simulink model "LF_AC29bus_HVDCdemo_V2_1"  (R2019b)
settings: Solver=FixedStepDiscrete  StartTime=0.0  StopTime=fix(6/Ts)*Ts  FixedStep=Ts  RelTol=1e-3
InitFcn:
  | Ts_avg=150e-6;
  | Ts=50e-6;
  | 
  | %Tc_stab = 1/60/5;
  | %Tc_stab = 2/60;
  | Tc_stab = Ts;
  | 
  | 
  | Ts_avg=150e-6;
  | 
  | Ts=50e-6;
  | 
  | % Rectifier AC side :
  | VLL_nom_R = 735e3; % V
  | Fnom_R = 60;           % Hz
  | 
  | % Inverter AC side :
  | VLL_nom_I = 735e3; % V
  | Fnom_I = 60;           % Hz
  | 
  | % DC :
  | Vdc_nom = 500e3;   % V
  | Idc_nom  = 2000;     % A
undefined symbols (not defined in the file): D1, D11, Delta, test_alpha
libraries: powerlib x223, powerlib_meascontrol x57, simulink x22, sps_avr x7
(part 2 of 10)

== system LF_AC29bus_HVDCdemo_V2_1/HVDC_network_avg ==
  note: HVDC 12-pulse Transmission System 1000 MW (500kV-2kA) 60 Hz (Average Model)
  Binv : powerlib/Measurements/Three-Phase V-I Measurement  VoltageMeasurement=phase-to-ground  SetLabelV=on  LabelV=Vabc_I  Vpu=on  VpuLL=off  CurrentMeasurement=yes  SetLabelI=on  LabelI=Iabc_I  Ipu=on  Pbase=100e6  Vbase=735e3  OutputType=Magnitude  PhasorSimulation=off  PSBequivalent=0
      settings: SourceProductName=Simscape Electrical
  Brect : powerlib/Measurements/Three-Phase V-I Measurement  VoltageMeasurement=phase-to-ground  SetLabelV=on  LabelV=Vabc_R  Vpu=on  VpuLL=off  CurrentMeasurement=yes  SetLabelI=on  LabelI=Iabc_R  Ipu=on  Pbase=100e6  Vbase=735e3  OutputType=Magnitude  PhasorSimulation=off  PSBequivalent=0
      settings: SourceProductName=Simscape Electrical
  DC line 800 km : powerlib/Elements/Distributed Parameters Line  Phases=1  Frequency=60  Resistance=0.015  Inductance=0.792e-3  Capacitance=14.4e-9  Length=800  x1=[-0.00275 0;-0.0027 0;-0.00265 0;-0.0026 0;-0.00255 0;-0.0025 0;-0.00245 0;-0.0024 0;-0.00235 0;-0.0023 0;-0.00225 0;-0.0022 0;-0.00215 0;-0.0021 0;-0.00205 0;-0.002 0;-0.00195 0;-0.0019 0;-0.00185 0;-0.0018 0;-0.00175 0;-0.0017 0;-0.00165 0;-0.0016 0;-0.00155 0;-0.0015 0;-0.00145 0;-0.0014 0;-0.00135 0;-0.0013 0;-0.00125 0;-0.0012 0;-0.00115 0;-0.0011 0;-0.00105 0;-0.001 0;-0.00095 0;-0.0009 0;-0.00085 0;-0.0008 0;-0.00075 0;-0.0007 0;-0.00065 0;-0.0006 0;-0.00055 0;-0.0005 0;-0.00045 0;-0.0004 0;-0.00035 0;-0.0003 0;-0.00025 0;-0.0002 0;-0.00015 0;-0.0001 0;-5e-05 0]  x2=[-0.00275 0;-0.0027 0;-0.00265 0;-0.0026 0;-0.00255 0;-0.0025 0;-0.00245 0;-0.0024 0;-0.00235 0;-0.0023 0;-0.00225 0;-0.0022 0;-0.00215 0;-0.0021 0;-0.00205 0;-0.002 0;-0.00195 0;-0.0019 0;-0.00185 0;-0.0018 0;-0.00175 0;-0.0017 0;-0.00165 0;-0.0016 0;-0.00155 0;-0.0015 0;-0.00145 0;-0.0014 0;-0.00135 0;-0.0013 0;-0.00125 0;-0.0012 0;-0.00115 0;-0.0011 0;-0.00105 0;-0.001 0;-0.00095 0;-0.0009 0;-0.00085 0;-0.0008 0;-0.00075 0;-0.0007 0;-0.00065 0;-0.0006 0;-0.00055 0;-0.0005 0;-0.00045 0;-0.0004 0;-0.00035 0;-0.0003 0;-0.00025 0;-0.0002 0;-0.00015 0;-0.0001 0;-5e-05 0]  x3=[-0.00275 0;-0.0027 0;-0.00265 0;-0.0026 0;-0.00255 0;-0.0025 0;-0.00245 0;-0.0024 0;-0.00235 0;-0.0023 0;-0.00225 0;-0.0022 0;-0.00215 0;-0.0021 0;-0.00205 0;-0.002 0;-0.00195 0;-0.0019 0;-0.00185 0;-0.0018 0;-0.00175 0;-0.0017 0;-0.00165 0;-0.0016 0;-0.00155 0;-0.0015 0;-0.00145 0;-0.0014 0;-0.00135 0;-0.0013 0;-0.00125 0;-0.0012 0;-0.00115 0;-0.0011 0;-0.00105 0;-0.001 0;-0.00095 0;-0.0009 0;-0.00085 0;-0.0008 0;-0.00075 0;-0.0007 0;-0.00065 0;-0.0006 0;-0.00055 0;-0.0005 0;-0.00045 0;-0.0004 0;-0.00035 0;-0.0003 0;-0.00025 0;-0.0002 0;-0.00015 0;-0.0001 0;-5e-05 0]  x4=[-0.00275 0;-0.0027 0;-0.00265 0;-0.0026 0;-0.00255 0;-0.0025 0;-0.00245 0;-0.0024 0;-0.00235 0;-0.0023 0;-0.00225 0;-0.0022 0;-0.00215 0;-0.0021 0;-0.00205 0;-0.002 0;-0.00195 0;-0.0019 0;-0.00185 0;-0.0018 0;-0.00175 0;-0.0017 0;-0.00165 0;-0.0016 0;-0.00155 0;-0.0015 0;-0.00145 0;-0.0014 0;-0.00135 0;-0.0013 0;-0.00125 0;-0.0012 0;-0.00115 0;-0.0011 0;-0.00105 0;-0.001 0;-0.00095 0;-0.0009 0;-0.00085 0;-0.0008 0;-0.00075 0;-0.0007 0;-0.00065 0;-0.0006 0;-0.00055 0;-0.0005 0;-0.00045 0;-0.0004 0;-0.00035 0;-0.0003 0;-0.00025 0;-0.0002 0;-0.00015 0;-0.0001 0;-5e-05 0]  x5=0.0027016794776583  V1=ones(3,3)  V2=ones(3,3)  I1=ones(3,3)  I2=ones(3,3)  nHarmo=1  Measurements=Phase-to-ground voltages
      settings: AttributesFormatString=\n  SourceProductName=Simscape Electrical
  Filters 60Hz1 : Subsystem
      mask Display: disp('AC filters \n60 Hz\n600 Mvar')
  Filters 60Hz2 : Subsystem
      mask Display: disp('AC filters \n60 Hz\n600 Mvar')
  Ground1 : powerlib/Elements/Ground  LConnTagsString=a
      settings: SourceProductName=Simscape Electrical
  Ground4 : powerlib/Elements/Ground  LConnTagsString=a
      settings: SourceProductName=Simscape Electrical
  Inverter Average model : Subsystem
  Inverter Control and Protection (Average model) : Subsystem
      mask Display: disp('Pole Control\n and Protection')
  Ld1 : powerlib/Elements/Series RLC Branch  LConnTagsString=__new0  RConnTagsString=__new0  BranchType=RL  Resistance=0.3  Inductance=0.5  SetiL0=off  InitialCurrent=0  Capacitance=1.0  Setx0=off  InitialVoltage=0  Measurements=None
      settings: AttributesFormatString=%<Resistance> (ohm), %<Inductance> (H)  SourceProductName=Simscape Electrical
  Ld2 : powerlib/Elements/Series RLC Branch  LConnTagsString=__new0  RConnTagsString=__new0  BranchType=RL  Resistance=0.3  Inductance=0.5  SetiL0=off  InitialCurrent=0  Capacitance=1.0  Setx0=off  InitialVoltage=0  Measurements=None
      settings: AttributesFormatString=%<Resistance> (ohm), %<Inductance> (H)  SourceProductName=Simscape Electrical
  Master Control : Subsystem
      mask Display: disp('Master Control')
  Rectifier Average model : Subsystem
  Rectifier Control and Protection (Average model) : Subsystem
      mask Display: disp('Pole Control\n and Protection')
  A : PMIOPort  Tag=PMCPort  Side=Left
  B : PMIOPort  Tag=PMCPort  Port=2  Side=Left
  C : PMIOPort  Tag=PMCPort  Port=3  Side=Left
  "A " : PMIOPort  Tag=PMCPort  Port=4  Side=Right
  "B " : PMIOPort  Tag=PMCPort  Port=5  Side=Right
  "C " : PMIOPort  Tag=PMCPort  Port=6  Side=Right
  connections:
  Ld2/RConn1 -- Inverter Average model/RConn1
  Ld1/RConn1 -- DC line 800 km/LConn1
  Ld1/LConn1 -- Rectifier Average model/RConn1
  Ld2/LConn1 -- DC line 800 km/RConn1
  Ground1/LConn1 -- Inverter Average model/RConn2
  Inverter Average model/LConn1 -- Binv/RConn1
  Inverter Average model/LConn2 -- Binv/RConn2
  Inverter Average model/LConn3 -- Binv/RConn3
  Brect/RConn1 -- Rectifier Average model/LConn1
  Brect/RConn2 -- Rectifier Average model/LConn2
  Brect/RConn3 -- Rectifier Average model/LConn3
  Rectifier Average model/RConn2 -- Ground4/LConn1
  Brect/LConn2 -- B/RConn1 -- Filters 60Hz1/LConn2
  Brect/LConn1 -- A/RConn1 -- Filters 60Hz1/LConn1
  Brect/LConn3 -- C/RConn1 -- Filters 60Hz1/LConn3
  "A "/RConn1 -- Binv/LConn1 -- Filters 60Hz2/LConn1
  "B "/RConn1 -- Binv/LConn2 -- Filters 60Hz2/LConn2
  "C "/RConn1 -- Binv/LConn3 -- Filters 60Hz2/LConn3

== system LF_AC29bus_HVDCdemo_V2_1/LG27_nodes ==
  Neutral : powerlib/Elements/Neutral  LConnTagsString=a  NodeNumber=4
      settings: SourceProductName=Simscape Electrical  SourceProductBaseCode=PS
  Neutral1 : powerlib/Elements/Neutral  LConnTagsString=a  NodeNumber=5
      settings: SourceProductName=Simscape Electrical  SourceProductBaseCode=PS
  Neutral2 : powerlib/Elements/Neutral  LConnTagsString=a  NodeNumber=6
      settings: SourceProductName=Simscape Electrical  SourceProductBaseCode=PS
  a : PMIOPort  Tag=PMCPort  Side=Left
  b : PMIOPort  Tag=PMCPort  Port=2  Side=Left
  c : PMIOPort  Tag=PMCPort  Port=3  Side=Left
  connections:
  c/RConn1 -- Neutral2/LConn1
  b/RConn1 -- Neutral1/LConn1
  a/RConn1 -- Neutral/LConn1

== system LF_AC29bus_HVDCdemo_V2_1/MTL Load ==
  note: Constant PQ
  note: Constant Z
  note: TOTAL LOAD = 15 500 MW
  22 000 MVA 735 kV/230 kV : powerlib/Elements/Three-Phase Transformer (Two Windings)  Winding1Connection=Yg  Winding2Connection=Delta (D1)  CoreType=Three single-phase transformers  SetSaturation=off  Hysteresis=off  DataFile='basic_model'  SetInitialFlux=off  Measurements=None  UNITS=pu  NominalPower=[ 22000e6 60 ]  Winding1="[ 735e3 0.002  0.12]"  Winding2=[230e3 0.002 0]  Rm=500  Lm=500  L0=0.5  Saturation="[ 0,0  ;  0.005,1.2  ;  1.0,1.4 ]"  InitialFluxes=[ 0.8 , -0.8 , 0.7 ]  BreakLoop=off  DiscreteSolver=Trapezoidal iterative  DataType=off  TransfoNumber=0
      settings: SourceProductName=Simscape Electrical
  230 kV/25 kV 18 000 MVA : powerlib/Elements/Three-Phase Transformer (Two Windings)  Winding1Connection=Yg  Winding2Connection=Delta (D1)  CoreType=Three single-phase transformers  SetSaturation=off  Hysteresis=off  DataFile='basic_model'  SetInitialFlux=off  Measurements=None  UNITS=pu  NominalPower=[18000e6 60 ]  Winding1="[ 230e3  0.08/30   0.08 ]"  Winding2="[ 25e3  0.08/30  0.08]"  Rm=500  Lm=500  L0=0.5  Saturation="[ 0,0  ;  0.005,1.2  ;  1.0,1.4 ]"  InitialFluxes=[ 0.8 , -0.8 , 0.7 ]  BreakLoop=off  DiscreteSolver=Trapezoidal iterative  DataType=off  TransfoNumber=0
      settings: SourceProductName=Simscape Electrical
  3500 MW : powerlib/Elements/Three-Phase Dynamic Load  NominalVoltage=[ 25e3 60 ]  ActiveReactivePowers=[3.5e+09 -2.66454e-07]  PositiveSequence=[1.013 -91.543]  ExternalControl=off  NpNq="[1.5  2.5]"  TimeConstants="[0  0  0  0]"  MinimumVoltage=0.7  Tfilter=1e-4  LoadFlowParameters=[4,0,0,0,0]
      settings: SourceProductName=Simscape Electrical  SourceProductBaseCode=PS
  ASM 25kV 5000MVA Pm=4000 MW : powerlib/Machines/Asynchronous Machine pu Units  RotorType=Squirrel-cage  PresetModel=No  MechanicalLoad=Torque Tm  ShowDetailedParameters=on  ReferenceFrame=Rotor  Units=pu  MeasurementBus=off  NominalParameters="[5000e6 25e3  60]"  Stator=[0.01117 0.04832]  Rotor=[0.006 0.04832]  Cage1=[0.01909 0.0397]  Cage2=[0.01909 0.0397]  Lm=2.424  Mechanical="[1  0   2]"  PolePairs=2  InitialConditions=[0.00500983 0 0.928577 0.928577 0.928577 -121.661 -241.661 -1.66098]  SimulateSaturation=off  Saturation="[0.212,0.4201,0.8125,1.0979,1.4799,2.2457,3.2586,4.5763,6.4763 ;   0.5,0.7,0.9,1,1.1,1.2 ,1.3,1.4,1.5]"  LoadFlowParameters=0  TsPowergui=0  TsBlock=-1  IterativeModel=Trapezoidal non iterative  IterativeDiscreteModel=Trapezoidal non iterative  Pmec=4000e6
      settings: SourceProductName=Simscape Electrical  SourceProductBaseCode=PS
  Load Flow Bus : powerlib/Measurements/Load Flow Bus  LConnTagsString=a  Phases=single  Connectors=on one side  ID=MTL2  Vbase=230e3  Vref=1  Vangle=0  VLF=1.03  VLFb=1  VLFc=1  angleLF=-53.86  angleLFb=0  angleLFc=0
      settings: AttributesFormatString=%<ID>\n%<Vbase>V\n%<VLF>pu\n%<angleLF>deg.  SourceProductName=Simscape Electrical
  Load Flow Bus1 : powerlib/Measurements/Load Flow Bus  LConnTagsString=a  Phases=single  Connectors=on one side  ID=MTL_25  Vbase=25e3  Vref=1  Vangle=0  VLF=1.013  VLFb=1  VLFc=1  angleLF=-91.54  angleLFb=0  angleLFc=0
      settings: AttributesFormatString=%<ID>\n%<Vbase>V\n%<VLF>pu\n%<angleLF>deg.  SourceProductName=Simscape Electrical
  MTL 2000 Mvar : powerlib/Elements/Three-Phase Parallel RLC Load  LConnTagsString=A|B|C  Configuration=Y (grounded)  NominalVoltage=25e3  Vabc=[1e3 1e3 1e3]  Vabcp=[1e3 1e3 1e3]  NominalFrequency=60  UnbalancedPower=off  ActivePower=0  InductivePower=0  CapacitivePower=2000e6  Pabc=[10e3 9e3 11e3]  QLabc=[100 90 110]  QCabc=[100 90 110]  Pabcp=[10e3 9e3 11e3]  QLabcp=[100 90 110]  QCabcp=[100 90 110]  Measurements=None  LoadType=constant Z
      settings: SourceProductName=Simscape Electrical
  MTL 3000 Mvar : powerlib/Elements/Three-Phase Parallel RLC Load  LConnTagsString=A|B|C  Configuration=Y (grounded)  NominalVoltage=230e3  Vabc=[1e3 1e3 1e3]  Vabcp=[1e3 1e3 1e3]  NominalFrequency=60  UnbalancedPower=off  ActivePower=0  InductivePower=0  CapacitivePower=3000e6  Pabc=[10e3 9e3 11e3]  QLabc=[100 90 110]  QCabc=[100 90 110]  Pabcp=[10e3 9e3 11e3]  QLabcp=[100 90 110]  QCabcp=[100 90 110]  Measurements=None  LoadType=constant Z
      settings: SourceProductName=Simscape Electrical
  MTL 4000 MW : powerlib/Elements/Three-Phase Parallel RLC Load  LConnTagsString=A|B|C  Configuration=Y (grounded)  NominalVoltage=(25000)*1.013  Vabc=[1e3 1e3 1e3]  Vabcp=[1e3 1e3 1e3]  NominalFrequency=60  UnbalancedPower=off  ActivePower=4000e6  InductivePower=0  CapacitivePower=0  Pabc=[10e3 9e3 11e3]  QLabc=[100 90 110]  QCabc=[100 90 110]  Pabcp=[10e3 9e3 11e3]  QLabcp=[100 90 110]  QCabcp=[100 90 110]  Measurements=None  LoadType=constant PQ
      settings: SourceProductName=Simscape Electrical
  "MTL 4000 MW  " : powerlib/Elements/Three-Phase Parallel RLC Load  LConnTagsString=A|B|C  Configuration=Y (grounded)  NominalVoltage=25e3  Vabc=[1e3 1e3 1e3]  Vabcp=[1e3 1e3 1e3]  NominalFrequency=60  UnbalancedPower=off  ActivePower=4000e6  InductivePower=0  CapacitivePower=0  Pabc=[10e3 9e3 11e3]  QLabc=[100 90 110]  QCabc=[100 90 110]  Pabcp=[10e3 9e3 11e3]  QLabcp=[100 90 110]  QCabcp=[100 90 110]  Measurements=None  LoadType=constant Z
      settings: SourceProductName=Simscape Electrical
  Terminator_1 : Terminator
  Terminator_2 : Terminator
  Tm : Constant  Value=0.80403
  A : PMIOPort  Side=Left
  B : PMIOPort  Port=2  Side=Left
  C : PMIOPort  Port=3  Side=Left
  wires:
  Tm/1 -> ASM 25kV 5000MVA Pm=4000 MW/1
  3500 MW/1 -> Terminator_1/1
  ASM 25kV 5000MVA Pm=4000 MW/1 -> Terminator_2/1
  connections:
  A/RConn1 -- 22 000 MVA 735 kV/230 kV/LConn1
  B/RConn1 -- 22 000 MVA 735 kV/230 kV/LConn2
  C/RConn1 -- 22 000 MVA 735 kV/230 kV/LConn3
  230 kV/25 kV 18 000 MVA/LConn1 -- Load Flow Bus/LConn1 -- 22 000 MVA 735 kV/230 kV/RConn1 -- MTL 3000 Mvar/LConn1
  230 kV/25 kV 18 000 MVA/LConn2 -- 22 000 MVA 735 kV/230 kV/RConn2 -- MTL 3000 Mvar/LConn2
  230 kV/25 kV 18 000 MVA/LConn3 -- 22 000 MVA 735 kV/230 kV/RConn3 -- MTL 3000 Mvar/LConn3
  ASM 25kV 5000MVA Pm=4000 MW/LConn1 -- MTL 2000 Mvar/LConn1 -- "MTL 4000 MW  "/LConn1 -- Load Flow Bus1/LConn1 -- MTL 4000 MW/LConn1 -- 230 kV/25 kV 18 000 MVA/RConn1 -- 3500 MW/LConn1
  ASM 25kV 5000MVA Pm=4000 MW/LConn2 -- MTL 2000 Mvar/LConn2 -- "MTL 4000 MW  "/LConn2 -- MTL 4000 MW/LConn2 -- 230 kV/25 kV 18 000 MVA/RConn2 -- 3500 MW/LConn2
  230 kV/25 kV 18 000 MVA/RConn3 -- ASM 25kV 5000MVA Pm=4000 MW/LConn3 -- MTL 2000 Mvar/LConn3 -- "MTL 4000 MW  "/LConn3 -- MTL 4000 MW/LConn3 -- 3500 MW/LConn3

== system LF_AC29bus_HVDCdemo_V2_1/MTL7_nodes ==
  Neutral : powerlib/Elements/Neutral  LConnTagsString=a  NodeNumber=1
      settings: SourceProductName=Simscape Electrical  SourceProductBaseCode=PS
  Neutral1 : powerlib/Elements/Neutral  LConnTagsString=a  NodeNumber=2
      settings: SourceProductName=Simscape Electrical  SourceProductBaseCode=PS
  Neutral2 : powerlib/Elements/Neutral  LConnTagsString=a  NodeNumber=3
      settings: SourceProductName=Simscape Electrical  SourceProductBaseCode=PS
  a : PMIOPort  Tag=PMCPort  Side=Left
  b : PMIOPort  Tag=PMCPort  Port=2  Side=Left
  c : PMIOPort  Tag=PMCPort  Port=3  Side=Left
  connections:
  a/RConn1 -- Neutral/LConn1
  b/RConn1 -- Neutral1/LConn1
  c/RConn1 -- Neutral2/LConn1

== system LF_AC29bus_HVDCdemo_V2_1/MTL7_nodes  ==
  Neutral : powerlib/Elements/Neutral  LConnTagsString=a  NodeNumber=1
      settings: SourceProductName=Simscape Electrical  SourceProductBaseCode=PS
  Neutral1 : powerlib/Elements/Neutral  LConnTagsString=a  NodeNumber=2
      settings: SourceProductName=Simscape Electrical  SourceProductBaseCode=PS
  Neutral2 : powerlib/Elements/Neutral  LConnTagsString=a  NodeNumber=3
      settings: SourceProductName=Simscape Electrical  SourceProductBaseCode=PS
  a : PMIOPort  Tag=PMCPort  Side=Left
  b : PMIOPort  Tag=PMCPort  Port=2  Side=Left
  c : PMIOPort  Tag=PMCPort  Port=3  Side=Left
  connections:
  c/RConn1 -- Neutral2/LConn1
  b/RConn1 -- Neutral1/LConn1
  a/RConn1 -- Neutral/LConn1
